simulink library "Teleop_lib"  (R2023b)
settings: Solver=VariableStepAuto  StartTime=0.0  StopTime=10.0  RelTol=1e-3
settings Model: Creator=FIRSTMentor  LastModifiedBy=USER

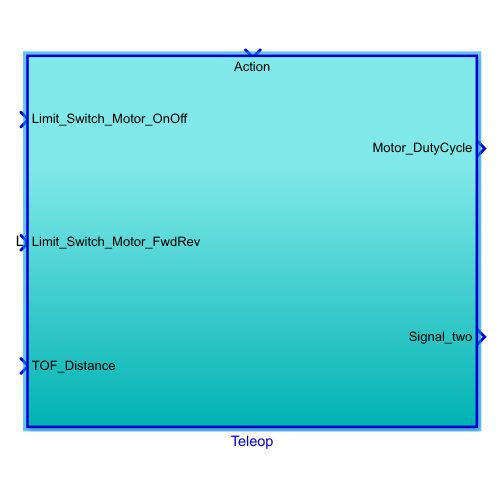
[thumbnail: Simulink's stored preview of the top-level diagram]
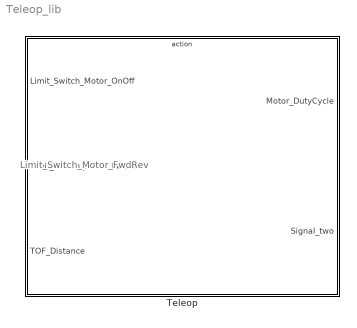
== system Teleop_lib ==
  note: Limit_Switch_Motor_FwdRev
  Teleop : Subsystem  TreatAsAtomicUnit=on

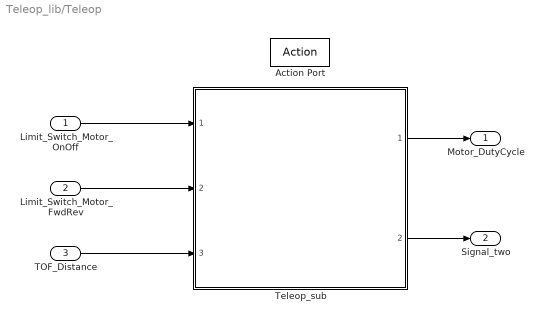
== system Teleop_lib/Teleop ==
  Limit_Switch_Motor_OnOff : Inport
  Limit_Switch_Motor_FwdRev : Inport  Port=2
  TOF_Distance : Inport  Port=3
  Action Port : ActionPort  InitializeStates=reset
  Teleop_sub : Subsystem  ReferencedSubsystem=Teleop_sub
  Motor_DutyCycle : Outport
  Signal_two : Outport  Port=2
  wires:
  Teleop_sub/1 -> Motor_DutyCycle/1
  Teleop_sub/2 -> Signal_two/1
  Limit_Switch_Motor_OnOff/1 -> Teleop_sub/1
  Limit_Switch_Motor_FwdRev/1 -> Teleop_sub/2
  TOF_Distance/1 -> Teleop_sub/3
